simulink model "HCM"  (R2019b)
settings: Solver=FixedStepDiscrete  StartTime=0.0  StopTime=inf  FixedStep=0.1  RelTol=1e-3
settings Model: Creator=JDALUZ1  LastModifiedBy=EMORAI12
settings SolverCC: PositivePriorityOrder=on  AutoInsertRateTranBlk=on  InsertRTBMode=Always
settings DebuggingCC: ArithmeticOperatorsInVariantConditions=warning
settings SFSimCC: CustomCodeUndefinedFunction=UseInterfaceOnly
settings CodeAppCC: StateflowObjectComments=on

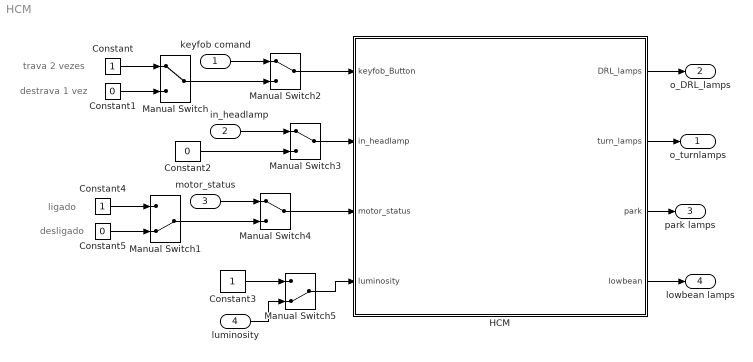
== system HCM ==
  note: destrava 1 vez
  note: trava 2 vezes
  note: ligado
  note: desligado
  keyfob comand : Inport
  in_headlamp : Inport  Port=2
  motor_status : Inport  Port=3
  luminosity : Inport  Port=4
  Constant : Constant
  Constant1 : Constant  Value=0
  Constant2 : Constant  Value=0
  Constant3 : Constant
  Constant4 : Constant
  Constant5 : Constant  Value=0
  HCM : Stateflow chart  TreatAsAtomicUnit=on
  Manual Switch{,2..4} (4 alike) : ManualSwitch
  Manual Switch1 : ManualSwitch  CurrentSetting=0
  Manual Switch5 : ManualSwitch  CurrentSetting=0
  o_turnlamps : Outport
  o_DRL_lamps : Outport  Port=2
  park lamps : Outport  Port=3  SignalName=park lamps
  lowbean lamps : Outport  Port=4  SignalName=lowbean lamps
  wires:
  Constant1/1 -> Manual Switch/2
  Constant/1 -> Manual Switch/1
  HCM/1(DRL_lamps) -> o_DRL_lamps/1
  HCM/2(turn_lamps) -> o_turnlamps/1
  Manual Switch2/1 -> HCM/1(keyfob_Button)
  Manual Switch/1 -> Manual Switch2/2
  keyfob comand/1 -> Manual Switch2/1
  in_headlamp/1 -> Manual Switch3/1
  Manual Switch3/1 -> HCM/2(in_headlamp)
  Constant2/1 -> Manual Switch3/2
  HCM/3(park) -> park lamps/1
  Constant4/1 -> Manual Switch1/1
  Manual Switch1/1 -> Manual Switch4/2
  Constant5/1 -> Manual Switch1/2
  motor_status/1 -> Manual Switch4/1
  Manual Switch4/1 -> HCM/3(motor_status)
  HCM/4(lowbean) -> lowbean lamps/1
  Constant3/1 -> Manual Switch5/1
  luminosity/1 -> Manual Switch5/2
  Manual Switch5/1 -> HCM/4(luminosity)

== stateflow chart HCM/HCM ==
  state stateGeral
    state Control_DRL_and_Turn_Lamps [parallel]
      settings: executionOrder=2
      state default
        entry:
        %o_headlamp=in_headlamp;
        turn_lamps=0; %turn_lamps desligadas
        r_aux=0;
        right_aux=0;
        left_aux=1;
        keyfob_Button_ant=keyfob_Button;
        during:
        %o_headlamp=in_headlamp;
        if(keyfob_Button_ant==keyfob_Button)
        keyfob_Button_ant=keyfob_Button;
        elseif(keyfob_Button_ant~=keyfob_Button)
        r_aux=1;
        end
      state Blinck_turn_lamps_twice
        entry:
        turn_lamps=1;
        during:
        left_aux=1;
        exit:
        DRL_lamps=0;
      state blinck_turn_lamps_once
        entry:
        turn_lamps=1;
        during:
        right_aux=1;
      state Blinck_turn_lamps_twice_off
        entry:
        turn_lamps=0;
        during:
        left_aux=2;
      state Turn_lamps_off
        entry:
        turn_lamps=0;
        during:
        right_aux=2;
      state Blinck_turn_lamps_twice_on
        entry:
        turn_lamps=1;
        during:
        left_aux=3;
      state DRL_ON
        entry:
        DRL_lamps=1;
        during:
        right_aux=3;
        exit:
        r_aux=0;
        down_aux=0;
      state Blinck_turn_lamps_twice1
        entry:
        turn_lamps=1;
        r_aux=0;
        during:
        left_aux=4;
        down_aux=0;
      (default) -> default
      default -> Blinck_turn_lamps_twice [order 2] : [keyfob_Button==0 && r_aux==1]
      default -> blinck_turn_lamps_once [order 1] : [keyfob_Button==1 &&r_aux==1]
      Blinck_turn_lamps_twice -> Blinck_turn_lamps_twice_off : [after(2,sec) && left_aux==1]
      blinck_turn_lamps_once -> Turn_lamps_off : [after(2,sec) && right_aux==1]
      Blinck_turn_lamps_twice1 -> default : [after(2,sec) && left_aux==4]
      DRL_ON -> default : [after(2,sec) && right_aux==3 ]
      Blinck_turn_lamps_twice_off -> Blinck_turn_lamps_twice_on : [after(2,sec) && left_aux==2]
      Turn_lamps_off -> DRL_ON : [after(2,sec) && right_aux==2]
      Blinck_turn_lamps_twice_on -> Blinck_turn_lamps_twice1 : [after(2,sec) && left_aux==3]
    state HEADLAMP_STATUS [parallel]
      entry:
      park=0;
      lowbean=0;
      during:
      if(in_headlamp==0)
      park=0;
      lowbean=0;
      elseif(in_headlamp==1)
      lowbean=0;
      park=1;
      elseif(in_headlamp==2)
      lowbean=1;
      park=0;
      elseif(in_headlamp==3)
      if(luminosity>=4) %muito claro
      lowbean=0;
      park=0;
      end
      if(luminosity>=2 && luminosity<4) %penumbra
      lowbean=0;
      park=1;
      end
      if(luminosity<=1) %penumbra
      lowbean=1;
      park=0;
      end
      end
      down_aux=1;
      settings: executionOrder=1
  (default) -> stateGeral
  data: DRL_lamps output; turn_lamps output; keyfob_Button input; keyfob_Button_ant local; r_aux local; in_headlamp input; right_aux local; left_aux local; down_aux local; park output; lowbean output; motor_status input; luminosity input
